simulink model "state_fdbk"  (R2019b)
settings: Solver=VariableStepAuto  StartTime=0.0  StopTime=120  RelTol=1e-3
values from neighbouring files (symbols this model uses):
  Dlong = 0    [model.m]
undefined symbols (not defined in the file or in its folder): Along_pl, Blong_pl, Clong_pl, K, L, Nbar
settings Model: Creator=brian  LastModifiedBy=brian

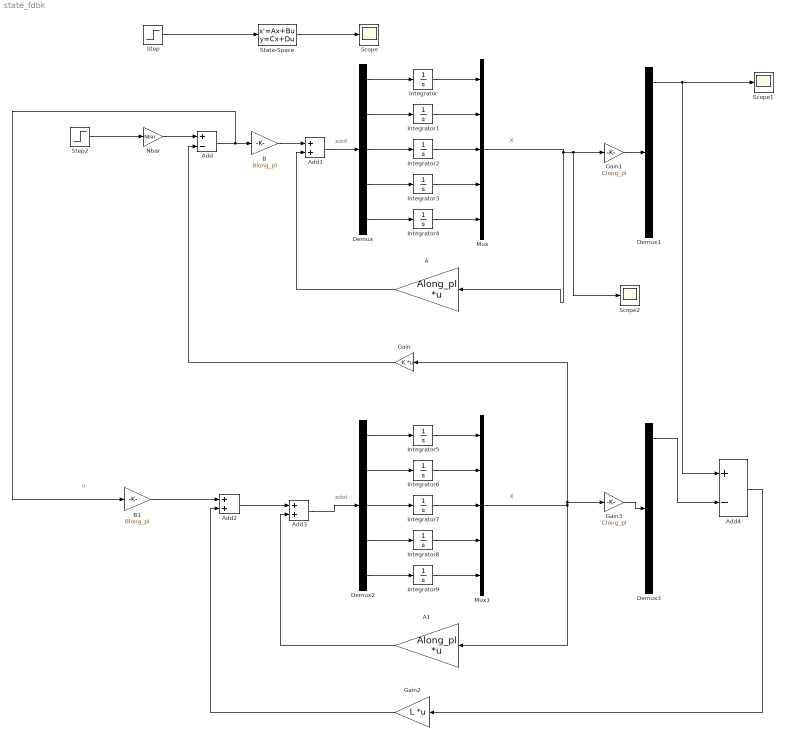
== system state_fdbk ==
  note: u
  note: xdot
  note: X
  note: xdot
  note: X
  A : Gain  Gain=Along_pl  Multiplication=Matrix(K*u)
  A1 : Gain  Gain=Along_pl  Multiplication=Matrix(K*u)
  Add : Sum  Inputs=+-
  Add1 : Sum
  Add2 : Sum
  Add3 : Sum
  Add4 : Sum  Inputs=+-
  B : Gain  Gain=Blong_pl
  B1 : Gain  Gain=Blong_pl
  Demux{,1..3} (4 alike) : Demux  Outputs=5
  Gain : Gain  Gain=K  Multiplication=Matrix(K*u)
  Gain1 : Gain  Gain=Clong_pl
  Gain2 : Gain  Gain=L  Multiplication=Matrix(K*u)
  Gain3 : Gain  Gain=Clong_pl
  Integrator{,1..9} (10 alike) : Integrator
  Mux : Mux  Inputs=5
  Mux1 : Mux  Inputs=5
  Nbar : Gain  Gain=Nbar
  Scope : Scope
  Scope1 : Scope
  Scope2 : Scope
  State-Space : StateSpace  A=Along_pl-Blong_pl*K  B=Blong_pl*Nbar  C=Clong_pl  D=Dlong  InitialCondition=0
  Step : Step  SampleTime=0
  Step2 : Step  After=-10  SampleTime=0
  wires:
  State-Space/1 -> Scope/1
  Step/1 -> State-Space/1
  Step2/1 -> Nbar/1
  Nbar/1 -> Add/1
  B/1 -> Add1/1
  Add1/1 -> Demux/1
  Demux/1 -> Integrator/1
  Demux/2 -> Integrator1/1
  Demux/3 -> Integrator2/1
  Demux/4 -> Integrator3/1
  Demux/5 -> Integrator4/1
  Integrator/1 -> Mux/1
  Integrator1/1 -> Mux/2
  Integrator2/1 -> Mux/3
  Integrator3/1 -> Mux/4
  Integrator4/1 -> Mux/5
  Mux/1 -> A/1, Scope2/1, Gain1/1
  A/1 -> Add1/2
  Gain/1 -> Add/2
  Gain1/1 -> Demux1/1
  Demux1/1 -> Add4/1, Scope1/1
  Integrator7/1 -> Mux1/3
  Demux2/2 -> Integrator6/1
  Demux2/1 -> Integrator5/1
  Integrator9/1 -> Mux1/5
  Gain3/1 -> Demux3/1
  Integrator8/1 -> Mux1/4
  Demux2/4 -> Integrator8/1
  Demux2/5 -> Integrator9/1
  A1/1 -> Add3/2
  Integrator5/1 -> Mux1/1
  Add/1 -> B1/1, B/1
  Add3/1 -> Demux2/1
  Integrator6/1 -> Mux1/2
  Demux2/3 -> Integrator7/1
  Demux3/1 -> Add4/2
  Add4/1 -> Gain2/1
  B1/1 -> Add2/1
  Gain2/1 -> Add2/2
  Add2/1 -> Add3/1
  Mux1/1 -> Gain/1, Gain3/1, A1/1
